simulink model "NLGC_4"  (R2017b)
settings: Solver=ode45  StartTime=0.0  StopTime=30  FixedStep=0.05  MaxStep=0.06  RelTol=1e-3  EnableMultiTasking=on
model workspace (MAT data in the model file):
  Sig = Simulink.Signal
  Sig.DataType = 'auto'
  Sig.Dimensions = -1
  Sig.DimensionsMode = 'auto'
  Sig.Complexity = 'auto'
  Sig.SampleTime = -1
  Sig.SamplingMode = 'auto'
undefined symbols (not defined in the file): IC, psi, quadModel, x, y, z
libraries: simulink x12, NLGCToolbox x11, sharedtransform x1
Description:
  | This is a configurable quadcopter simulation.
  | This Simulink model demonstates position control.
  | 
  | Additional quadcopter modeling and simulation materials available at:
  | github.com/dch33/Quad-Sim
  | 
  | Copyright (C) 2014 D. Hartman, K. Landis, S. Moreno, J. Kim, M. Mehrer
  | 
  | License:
  |     This program is free software: you can redistribute it and/or modify
  |     it under the terms of the GNU LESSER GENERAL PUBLIC LICENSE as published by
  |     the Free Software Foundation, either version 3 of the License, or
  |     (at your option) any later version.
  | 
  |     This program is distributed in the hope that it will be useful,
  |     but WITHOUT ANY WARRANTY; without even the implied warranty of
  |     MERCHANTABILITY or FITNESS FOR A PARTICULAR PURPOSE.  See the
  |     GNU General Public License for more details.
  | 
  |     You should have received a copy of the GNU LESSER GENERAL PUBLIC LICENSE
  |     along with this program.  If not, see <http://www.gnu.org/licenses/>.
settings Model: ModifiedComment=hoang -- Wed Apr 11 06:13:36 2018 -- Version 1.7  Creator=David Hartman  LastModifiedBy=hoang
settings Model: ModifiedHistory=|
  | hoang -- Wed Apr 11 06:13:36 2018 -- Version 1.7
  | 
  | hoang -- Wed Apr 11 04:36:33 2018 -- Version 1.6
  | 
  | davidhartman -- Fri Jun 06 22:59:54 2014 -- Version 1.5
settings DataIOCC: SaveFormat=Array  SignalLogging=off
settings OptimizationCC: DefaultParameterBehavior=Inlined  LifeSpan=inf
settings DebuggingCC: SolverPrmCheckMsg=warning  UniqueDataStoreMsg=warning  StateNameClashWarn=warning  StrictBusMsg=ErrorOnBusTreatedAsVector  SFUnexpectedBacktrackingDiag=warning  SFNoUnconditionalDefaultTransitionDiag=warning  SFExecutionAtInitializationDiag=none
settings HardwareCC: ProdBitPerPointer=32  ProdBitPerSizeT=32  ProdBitPerPtrDiffT=32  ProdLargestAtomicFloat=None  ProdIntDivRoundTo=Undefined  ProdEndianess=Unspecified  ProdWordSize=32  ProdHWDeviceType=32-bit Generic
settings ModelReferenceCC: PropagateSignalLabelsOutOfModel=off
settings CodeAppCC: StateflowObjectComments=on
settings GRTTargetCC: TargetLangStandard=C89/C90 (ANSI)  GeneratePreprocessorConditionals=Disable all
settings ConfigComp: CovMetricSettings=dw  CovHtmlReporting=on  CovSaveCumulativeToWorkspaceVar=on  CovSaveSingleToWorkspaceVar=on  CovExternalEMLEnable=off

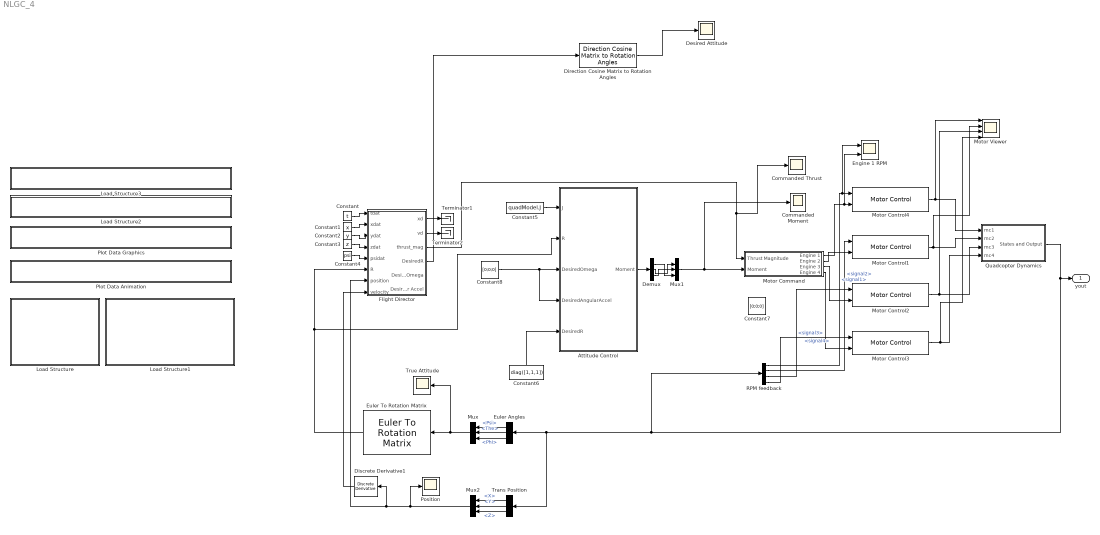
== system NLGC_4 ==
  Attitude Control : Subsystem  AncestorBlock=NLGCToolbox/Attitude Control  mask{kr=96, ko=1.25, Ts=1/60}
      mask prompts: kr "Attitude error gain (Kr)"; ko "Angular velocity error gain (Ko)"; Ts "Sampling Time (Ts)"
      mask init:
      | set_param(gcb, 'MaskSelfModifiable', 'on');
      settings: OpenFcn=set_param(gcbh,'LinkStatus','none');
  Commanded Thrust : Scope
  Commanded Moment : Scope
  Constant : Constant  Value=t
  Constant1 : Constant  Value=x
  Constant2 : Constant  Value=y
  Constant3 : Constant  Value=z
  Constant4 : Constant  Value=psi
  Constant5 : Constant  Value=quadModel.J
  Constant6 : Constant  Value=diag([1,1,1])
  Constant7 : Constant  Value=[0;0;0]
  Constant8 : Constant  Value=[0;0;0]
  Demux : Demux  Outputs=3
  Desired Attitude : Scope
  Direction Cosine Matrix to Rotation Angles : sharedtransform/Direction Cosine Matrix to Rotation Angles  rotationOrder=XYZ
      settings: SourceProductName=Aerospace Blockset  SourceProductBaseCode=AE
  Discrete Derivative1 : simulink/Discrete/Discrete Derivative  gainval=1.0  ICPrevScaledInput=[IC.X;IC.Y;IC.Z]*60  OutMin=[]  OutMax=[]  OutDataType=fixdt(1, 16)  OutScaling=2^-10  DoSatur=off
  Engine 1 RPM : Scope  NumInputPorts=2
  Euler Angles : BusSelector  OutputSignals=Psi,The,Phi
  Euler To Rotation Matrix : NLGCToolbox/Euler To Rotation Matrix
      settings: SourceProductName=Thinh - NLGC for Quadrotor
  Flight Director : Subsystem  AncestorBlock=NLGCToolbox/Flight Director  mask{Ts=1/60, kx=16, kv=5.6}
      mask prompts: Ts "Sampling Time (Ts)"; kx "Position Control Gain (kx)"; kv "Velocity Control Gain (kv)"
      settings: OpenFcn=set_param(gcbh,'LinkStatus','none');
  Load Structure : Subsystem
      settings: OpenFcn=|
      | uiopen('load')
      | if ((exist('IC')==1) && (exist('quadModel')==1) && (exist('path')==1))
      | set_param(bdroot, 'SimulationCommand', 'update')
      | end
      mask Display: fprintf('LOAD:\nTimeseries\nPath\nCommands,\nQuadcopter\nModel, Or\nInitial\nConditions');
  Load Structure1 : Subsystem
      settings: OpenFcn=|
      | if (exist('IC')==1 && exist('quadModel')==1 && exist('yout') && exist('tout'))
      | saveSimResults()
      | else
      | msgbox('No Data To Save!')
      | end
      mask Display: fprintf('SAVE:\nSimulation\nResults');
  Load Structure2 : Subsystem
      settings: OpenFcn=|
      | if exist('GUI_Modeling') == 2,
      | run('GUI_Modeling')
      | 
      | else
      | 
      | msgbox('The desired GUI must be first added to MATLABs path.')
      | 
      | end
      mask Display: fprintf('OPEN GUI: Build New \n Model');
  Load Structure3 : Subsystem
      settings: OpenFcn=|
      | if exist('GUI_IC') == 2,
      | run('GUI_IC')
      | 
      | else
      | 
      | msgbox('The desired GUI must be first added to MATLABs path.')
      | 
      | end
      mask Display: fprintf('OPEN GUI: Create Initial \n Conditions');
  Motor Command : Subsystem  AncestorBlock=NLGCToolbox/Motor Command  mask{Ct=quadModel.ct, dctcq=quadModel.dctcq}
      mask prompts: Ct "Force coefficient (Ct)"; dctcq "Moment coefficients matrix (dctcq)"
      settings: OpenFcn=set_param(gcbh,'LinkStatus','none');
  Motor Control{1..4} (4 alike) : NLGCToolbox/Motor Control  k=2.26  Km=quadModel.cr  Ts=1/60  T=quadModel.T  Rdt=100  Rdx=2  b=quadModel.b
      settings: SourceProductName=Thinh - NLGC for Quadrotor
  Motor Viewer : Scope  NumInputPorts=4
  Mux : Mux  Inputs=3
  Mux1 : Mux  Inputs=3
  Mux2 : Mux  Inputs=3
  Plot Data Animation : Subsystem
      settings: OpenFcn=|
      | if exist('QuadAnim4') == 2,
      |     if exist('yout')
      | 	run('QuadAnim4');
      |     else
      |     msgbox('Simulation must be run before data can be plotted.');
      |     end
      | else                                                                          msgbox('The desired GUI must be first added to MATLABs path.')
      | end
      mask Display: fprintf('OPEN GUI: Flight Animation')
  Plot Data Graphics : Subsystem
      settings: OpenFcn=|
      | if exist('yout')
      | yout = evalin('base', 'yout');
      | tout = evalin('base', 'tout');
      | quadPlots(yout, tout)
      | else
      | msgbox('Simulation must be run before data can be plotted.')
      | end
      mask Display: fprintf('OPEN PLOT: State Data')
  Position : Scope
  Quadcopter Dynamics : Subsystem
  RPM feedback : BusSelector  OutputSignals=mc and RPM.signal1,mc and RPM.signal2,mc and RPM.signal3,mc and RPM.signal4
  Terminator1 : Terminator
  Terminator2 : Terminator
  Trans Position : BusSelector  OutputSignals=X,Y,Z
  True Attitude : Scope
  yout : Outport
  wires:
  Quadcopter Dynamics/1(States and Output) -> RPM feedback/1, Trans Position/1, Euler Angles/1, yout/1
  Mux/1 -> Euler To Rotation Matrix/1, True Attitude/1
  Trans Position/3 -> Mux2/3  "<Z>"
  Mux2/1 -> Position/1, Flight Director/7(position), Discrete Derivative1/1
  Constant5/1 -> Attitude Control/1(J)
  Flight Director/3(thrust_mag) -> Motor Command/1(" Thrust Magnitude"), Commanded Thrust/1
  Motor Command/1(Engine 1) -> Motor Control4/2, Engine 1 RPM/2
  Motor Command/2(Engine 2) -> Motor Control1/2
  Motor Command/3(Engine 3) -> Motor Control2/2
  Motor Command/4(Engine 4) -> Motor Control3/2
  Motor Control4/1 -> Motor Viewer/1, Quadcopter Dynamics/1(mc1)
  Motor Control1/1 -> Motor Viewer/2, Quadcopter Dynamics/2(mc2)
  Motor Control3/1 -> Motor Viewer/4, Quadcopter Dynamics/4(mc4)
  RPM feedback/1 -> Motor Control4/1, Engine 1 RPM/1  "<signal1>"
  RPM feedback/2 -> Motor Control1/1  "<signal2>"
  RPM feedback/3 -> Motor Control2/1  "<signal3>"
  RPM feedback/4 -> Motor Control3/1  "<signal4>"
  Constant/1 -> Flight Director/1(tdat)
  Constant1/1 -> Flight Director/2(xdat)
  Discrete Derivative1/1 -> Flight Director/8(velocity)
  Direction Cosine Matrix to Rotation Angles/1 -> Desired Attitude/1
  Motor Control2/1 -> Motor Viewer/3, Quadcopter Dynamics/3(mc3)
  Trans Position/2 -> Mux2/2  "<Y>"
  Trans Position/1 -> Mux2/1  "<X>"
  Euler Angles/1 -> Mux/1  "<Psi>"
  Euler Angles/2 -> Mux/2  "<The>"
  Euler Angles/3 -> Mux/3  "<Phi>"
  Flight Director/4(DesiredR) -> Direction Cosine Matrix to Rotation Angles/1
  Constant2/1 -> Flight Director/3(ydat)
  Constant3/1 -> Flight Director/4(zdat)
  Constant4/1 -> Flight Director/5(psidat)
  Flight Director/1(xd) -> Terminator1/1
  Flight Director/2(vd) -> Terminator2/1
  Attitude Control/1(Moment) -> Demux/1
  Mux1/1 -> Commanded Moment/1, Motor Command/2(Moment)
  Constant8/1 -> Attitude Control/4(DesiredAngularAccel), Attitude Control/3(DesiredOmega)
  ? -> ?
  Euler To Rotation Matrix/1 -> Attitude Control/2(R), Flight Director/6(R)
  Constant6/1 -> Attitude Control/5(DesiredR)
  Demux/1 -> Mux1/3
  Demux/3 -> Mux1/1
  Demux/2 -> Mux1/2

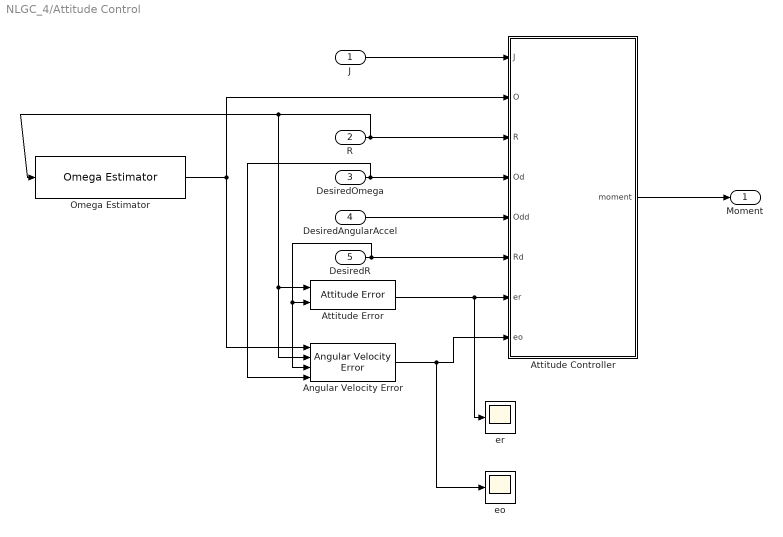
== system NLGC_4/Attitude Control ==
  J : Inport
  R : Inport  Port=2
  DesiredOmega : Inport  Port=3
  DesiredAngularAccel : Inport  Port=4
  DesiredR : Inport  Port=5
  Angular Velocity Error : NLGCToolbox/Angular Velocity Error
      settings: SourceProductName=Thinh - NLGC for Quadrotor
  Attitude Controller : MATLAB Function  TreatAsAtomicUnit=on
  Attitude Error : NLGCToolbox/Attitude Error
      settings: SourceProductName=Thinh - NLGC for Quadrotor
  Omega Estimator : NLGCToolbox/Omega Estimator  Ts=Ts
      settings: SourceProductName=Thinh - NLGC for Quadrotor
  eo : Scope
  er : Scope
  Moment : Outport
  wires:
  Angular Velocity Error/1 -> eo/1, Attitude Controller/8(eo)
  Attitude Error/1 -> er/1, Attitude Controller/7(er)
  J/1 -> Attitude Controller/1(J)
  Omega Estimator/1 -> Angular Velocity Error/1, Attitude Controller/2(O)
  R/1 -> Attitude Controller/3(R), Omega Estimator/1, Attitude Error/1, Angular Velocity Error/2
  DesiredOmega/1 -> Attitude Controller/4(Od), Angular Velocity Error/4
  DesiredAngularAccel/1 -> Attitude Controller/5(Odd)
  DesiredR/1 -> Attitude Controller/6(Rd), Attitude Error/2, Angular Velocity Error/3
  Attitude Controller/1(moment) -> Moment/1

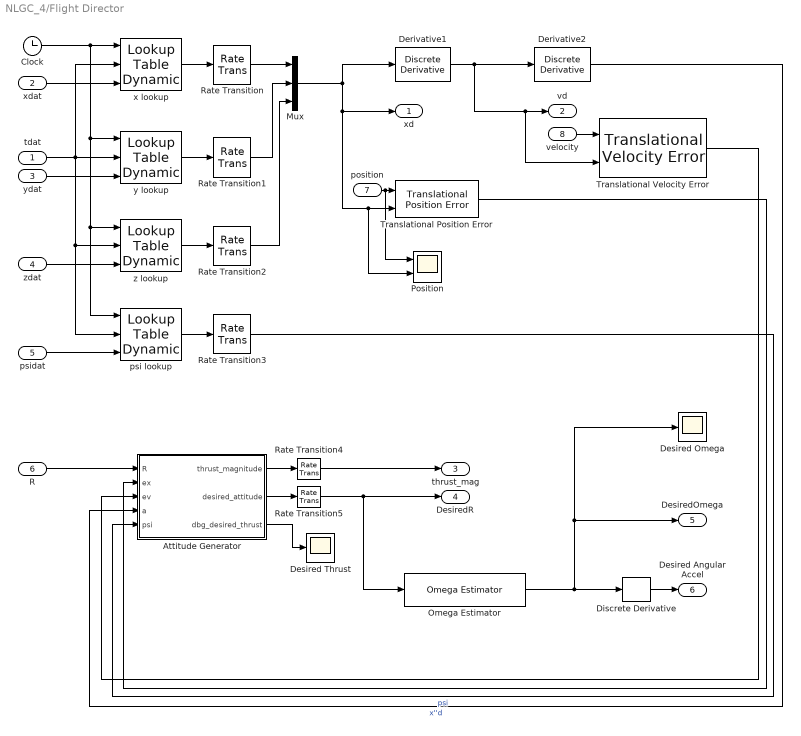
== system NLGC_4/Flight Director ==
  tdat : Inport
  xdat : Inport  Port=2
  ydat : Inport  Port=3
  zdat : Inport  Port=4
  psidat : Inport  Port=5
  R : Inport  Port=6
  position : Inport  Port=7
  velocity : Inport  Port=8
  Attitude Generator : MATLAB Function  TreatAsAtomicUnit=on
  Clock : Clock
  Derivative1 : simulink/Discrete/Discrete Derivative  gainval=1.0  ICPrevScaledInput=[0;0;3]*60  OutMin=[]  OutMax=[]  OutDataType=fixdt(1, 16)  OutScaling=2^-10  DoSatur=off
  Derivative2 : simulink/Discrete/Discrete Derivative  gainval=1.0  ICPrevScaledInput=0.0  OutMin=[]  OutMax=[]  OutDataType=fixdt(1, 16)  OutScaling=2^-10  DoSatur=off
  Desired Omega : Scope
  Desired Thrust : Scope
  Discrete Derivative : simulink/Discrete/Discrete Derivative  gainval=1.0  ICPrevScaledInput=0.0  OutMin=[]  OutMax=[]  OutDataType=fixdt(1, 16)  OutScaling=2^-10  DoSatur=off
  Mux : Mux  Inputs=3
  Omega Estimator : NLGCToolbox/Omega Estimator  Ts=Ts
      settings: SourceProductName=Thinh - NLGC for Quadrotor
  Position : Scope  NumInputPorts=2
  Rate Transition{,1..5} (6 alike) : RateTransition  OutPortSampleTime=Ts
  Translational Position Error : NLGCToolbox/Translational Position Error
      settings: SourceProductName=Thinh - NLGC for Quadrotor
  Translational Velocity Error : NLGCToolbox/Translational Velocity Error
      settings: SourceProductName=Thinh - NLGC for Quadrotor
  psi lookup : simulink/Lookup Tables/Lookup Table Dynamic  LookUpMeth=Interpolation-Use End Values  OutDataType=fixdt('double')  OutScaling=[]  OutputDataTypeScalingMode=Specify via dialog  OutDataTypeStr=double  DoSatur=off
      settings: SourceProductName=Simulink
  x lookup : simulink/Lookup Tables/Lookup Table Dynamic  LookUpMeth=Interpolation-Use End Values  OutDataType=fixdt('double')  OutScaling=[]  OutputDataTypeScalingMode=Specify via dialog  OutDataTypeStr=double  DoSatur=off
      settings: SourceProductName=Simulink
  y lookup : simulink/Lookup Tables/Lookup Table Dynamic  LookUpMeth=Interpolation-Use End Values  OutDataType=fixdt('double')  OutScaling=[]  OutputDataTypeScalingMode=Specify via dialog  OutDataTypeStr=double  DoSatur=off
      settings: SourceProductName=Simulink
  z lookup : simulink/Lookup Tables/Lookup Table Dynamic  LookUpMeth=Interpolation-Use End Values  OutDataType=fixdt('double')  OutScaling=[]  OutputDataTypeScalingMode=Specify via dialog  OutDataTypeStr=double  DoSatur=off
      settings: SourceProductName=Simulink
  xd : Outport
  vd : Outport  Port=2
  thrust_mag : Outport  Port=3
  DesiredR : Outport  Port=4
  DesiredOmega : Outport  Port=5
  Desired Angular Accel : Outport  Port=6
  wires:
  Omega Estimator/1 -> Discrete Derivative/1, DesiredOmega/1, Desired Omega/1
  velocity/1 -> Translational Velocity Error/1
  psidat/1 -> psi lookup/3
  Translational Velocity Error/1 -> Attitude Generator/3(ev)
  Translational Position Error/1 -> Attitude Generator/2(ex)
  Mux/1 -> Derivative1/1, Position/2, Translational Position Error/2, xd/1
  Rate Transition4/1 -> thrust_mag/1
  Rate Transition5/1 -> DesiredR/1, Omega Estimator/1
  Discrete Derivative/1 -> Desired Angular Accel/1
  R/1 -> Attitude Generator/1(R)
  Attitude Generator/2(desired_attitude) -> Rate Transition5/1
  Attitude Generator/1(thrust_magnitude) -> Rate Transition4/1
  Rate Transition3/1 -> Attitude Generator/5(psi)  "psi"
  Derivative2/1 -> Attitude Generator/4(a)  "x''d"
  psi lookup/1 -> Rate Transition3/1
  Derivative1/1 -> Derivative2/1, vd/1, Translational Velocity Error/2
  Rate Transition2/1 -> Mux/3
  Rate Transition1/1 -> Mux/2
  Rate Transition/1 -> Mux/1
  z lookup/1 -> Rate Transition2/1
  y lookup/1 -> Rate Transition1/1
  x lookup/1 -> Rate Transition/1
  zdat/1 -> z lookup/3
  ydat/1 -> y lookup/3
  xdat/1 -> x lookup/3
  Clock/1 -> x lookup/1, y lookup/1, z lookup/1, psi lookup/1
  tdat/1 -> y lookup/2, x lookup/2, z lookup/2, psi lookup/2
  Attitude Generator/3(dbg_desired_thrust) -> Desired Thrust/1
  position/1 -> Position/1, Translational Position Error/1

== system NLGC_4/Load Structure ==

== system NLGC_4/Load Structure1 ==

== system NLGC_4/Load Structure2 ==

== system NLGC_4/Load Structure3 ==

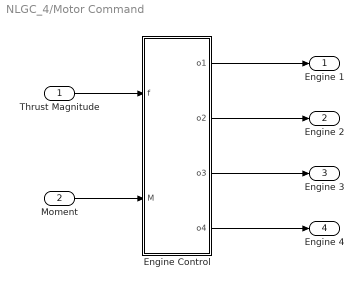
== system NLGC_4/Motor Command ==
  " Thrust Magnitude" : Inport
  Moment : Inport  Port=2
  Engine Control : MATLAB Function  TreatAsAtomicUnit=on
  Engine 1 : Outport
  Engine 2 : Outport  Port=2
  Engine 3 : Outport  Port=3
  Engine 4 : Outport  Port=4
  wires:
  Engine Control/4(o4) -> Engine 4/1
  Engine Control/3(o3) -> Engine 3/1
  Engine Control/2(o2) -> Engine 2/1
  Engine Control/1(o1) -> Engine 1/1
  Moment/1 -> Engine Control/2(M)
  " Thrust Magnitude"/1 -> Engine Control/1(f)

== system NLGC_4/Plot Data Animation ==

== system NLGC_4/Plot Data Graphics ==

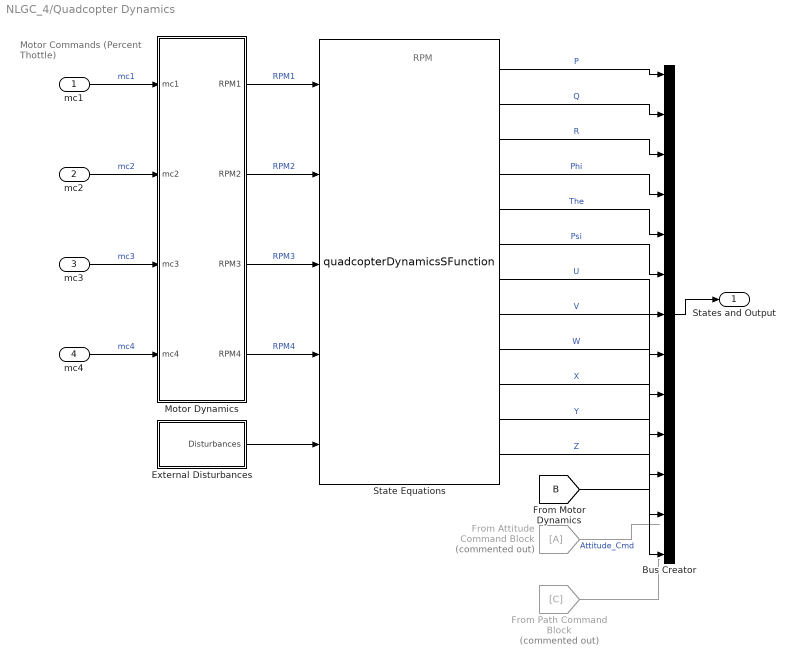
== system NLGC_4/Quadcopter Dynamics ==
  note: RPM
  note: Motor Commands
      | (Percent Thottle)
  mc1 : Inport
  mc2 : Inport  Port=2
  mc3 : Inport  Port=3
  mc4 : Inport  Port=4
  Bus Creator : BusCreator  Inputs=P,Q,R,Phi,The,Psi,U,V,W,X,Y,Z,mc and RPM
  External Disturbances : Subsystem
  From Attitude Command Block : From  Commented=on  TagVisibility=global
  From Path Command Block : From  Commented=on  GotoTag=C  TagVisibility=global
  Motor Dynamics : Subsystem
  State Equations : M-S-Function  FunctionName=quadcopterDynamicsSFunction  Parameters=quadModel, IC
      mask Display:
      | port_label('input', 1, 'RPM1')
      | port_label('input', 2, 'RPM2')
      | port_label('input', 3, 'RPM3')
      | port_label('input', 4, 'RPM4')
      | port_label('input', 5, 'Disturbances')
      | port_label('output', 1, 'P')
      | port_label('output', 2, 'Q')
      | port_label('output', 3, 'R')
      | port_label('output', 4, 'Phi')
      | port_label('output', 5, 'The')
      | port_label('output', 6, 'Psi')
      | port_label('output', 7, 'U')
      | port_label('output', 8, 'V')
      | port_label('output', 9, 'W')
      | port_label('output', 10, 'X')
      | port_label('output', 11, 'Y')
      | port_label('output', 12, 'Z')
  States and Output : Outport
  wires:
  State Equations/1 -> Bus Creator/1  "P"
  State Equations/2 -> Bus Creator/2  "Q"
  State Equations/3 -> Bus Creator/3  "R"
  State Equations/4 -> Bus Creator/4  "Phi"
  State Equations/5 -> Bus Creator/5  "The"
  State Equations/6 -> Bus Creator/6  "Psi"
  State Equations/7 -> Bus Creator/7  "U"
  State Equations/8 -> Bus Creator/8  "V"
  State Equations/9 -> Bus Creator/9  "W"
  State Equations/10 -> Bus Creator/10  "X"
  State Equations/11 -> Bus Creator/11  "Y"
  State Equations/12 -> Bus Creator/12  "Z"
  Bus Creator/1 -> States and Output/1
  Motor Dynamics/1(RPM1) -> State Equations/1  "RPM1"
  Motor Dynamics/2(RPM2) -> State Equations/2  "RPM2"
  Motor Dynamics/3(RPM3) -> State Equations/3  "RPM3"
  Motor Dynamics/4(RPM4) -> State Equations/4  "RPM4"
  mc1/1 -> Motor Dynamics/1(mc1)  "mc1"
  mc4/1 -> Motor Dynamics/4(mc4)  "mc4"
  mc3/1 -> Motor Dynamics/3(mc3)  "mc3"
  mc2/1 -> Motor Dynamics/2(mc2)  "mc2"
  External Disturbances/1("Disturbances ") -> State Equations/5
  From Attitude Command Block/1 -> ?  "Attitude_Cmd"
  [B] -> Bus Creator/13
  From Path Command Block/1 -> ?

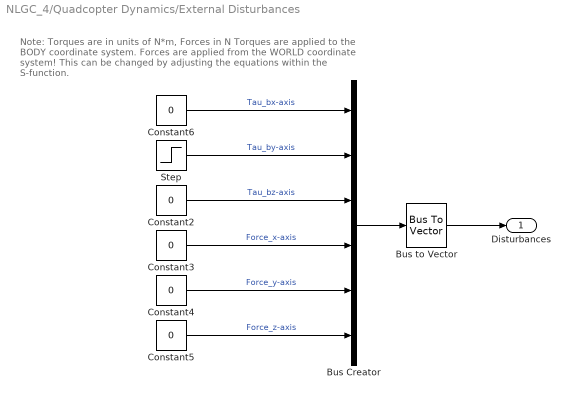
== system NLGC_4/Quadcopter Dynamics/External Disturbances ==
  note: Note: Torques are in units of N*m, Forces in N
      | Torques are applied to the BODY coordinate system.
      | Forces are applied from the WORLD coordinate system!
      | This can be changed by adjusting the equations within the S-function.
  Bus Creator : BusCreator  Inputs=6
  Bus to Vector : BusToVector
  Constant{2..6} (5 alike) : Constant  Value=0
  Step : Step  After=0  SampleTime=0
  "Disturbances " : Outport
  wires:
  Bus to Vector/1 -> "Disturbances "/1
  Bus Creator/1 -> Bus to Vector/1
  Constant6/1 -> Bus Creator/1  "Tau_bx-axis"
  Step/1 -> Bus Creator/2  "Tau_by-axis"
  Constant2/1 -> Bus Creator/3  "Tau_bz-axis"
  Constant3/1 -> Bus Creator/4  "Force_x-axis"
  Constant4/1 -> Bus Creator/5  "Force_y-axis"
  Constant5/1 -> Bus Creator/6  "Force_z-axis"

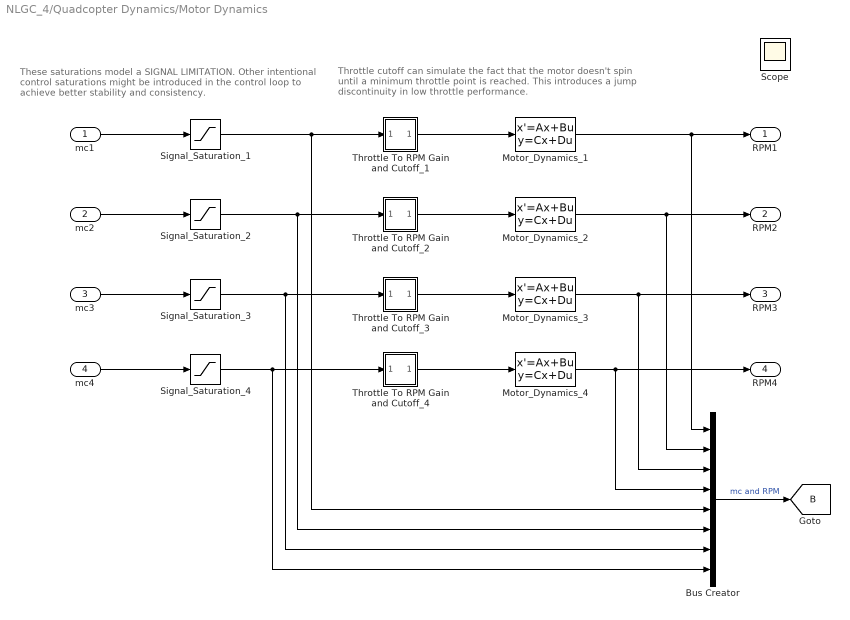
== system NLGC_4/Quadcopter Dynamics/Motor Dynamics ==
  note: Throttle cutoff can simulate the fact that the motor doesn't
      | spin until a minimum throttle point is reached. This introduces
      | a jump discontinuity in low throttle performance.
  note: These saturations model a SIGNAL LIMITATION.
      | Other intentional control saturations might be introduced in the
      | control loop to achieve better stability and consistency.
  mc1 : Inport
  mc2 : Inport  Port=2
  mc3 : Inport  Port=3
  mc4 : Inport  Port=4
  Bus Creator : BusCreator  Inputs=8
  Motor_Dynamics_1 : StateSpace  A=-1/quadModel.T  C=1/quadModel.T  D=0  InitialCondition=IC.w1*quadModel.T
  Motor_Dynamics_2 : StateSpace  A=-1/quadModel.T  C=1/quadModel.T  D=0  InitialCondition=IC.w2*quadModel.T
  Motor_Dynamics_3 : StateSpace  A=-1/quadModel.T  C=1/quadModel.T  D=0  InitialCondition=IC.w3*quadModel.T
  Motor_Dynamics_4 : StateSpace  A=-1/quadModel.T  C=1/quadModel.T  D=0  InitialCondition=IC.w4*quadModel.T
  Scope : Scope
  Signal_Saturation_{1..4} (4 alike) : Saturate  UpperLimit=100  LowerLimit=0
  Throttle To RPM Gain and Cutoff_1 : Subsystem
  Throttle To RPM Gain and Cutoff_2 : Subsystem
  Throttle To RPM Gain and Cutoff_3 : Subsystem
  Throttle To RPM Gain and Cutoff_4 : Subsystem
  RPM1 : Outport
  RPM2 : Outport  Port=2
  RPM3 : Outport  Port=3
  RPM4 : Outport  Port=4
  tag scope: B=global
  wires:
  mc1/1 -> Signal_Saturation_1/1
  mc4/1 -> Signal_Saturation_4/1
  mc2/1 -> Signal_Saturation_2/1
  mc3/1 -> Signal_Saturation_3/1
  Signal_Saturation_1/1 -> Bus Creator/5, Throttle To RPM Gain and Cutoff_1/1(In5)
  Signal_Saturation_2/1 -> Bus Creator/6, Throttle To RPM Gain and Cutoff_2/1(In5)
  Signal_Saturation_3/1 -> Bus Creator/7, Throttle To RPM Gain and Cutoff_3/1(In5)
  Signal_Saturation_4/1 -> Bus Creator/8, Throttle To RPM Gain and Cutoff_4/1(In5)
  Throttle To RPM Gain and Cutoff_1/1(Out5) -> Motor_Dynamics_1/1
  Throttle To RPM Gain and Cutoff_2/1(Out5) -> Motor_Dynamics_2/1
  Throttle To RPM Gain and Cutoff_3/1(Out5) -> Motor_Dynamics_3/1
  Throttle To RPM Gain and Cutoff_4/1(Out5) -> Motor_Dynamics_4/1
  Motor_Dynamics_1/1 -> Bus Creator/1, RPM1/1
  Motor_Dynamics_2/1 -> Bus Creator/2, RPM2/1
  Motor_Dynamics_3/1 -> Bus Creator/3, RPM3/1
  Motor_Dynamics_4/1 -> Bus Creator/4, RPM4/1
  Bus Creator/1 -> [B]  "mc and RPM"

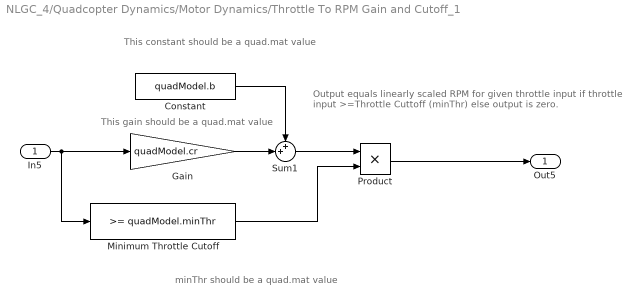
== system NLGC_4/Quadcopter Dynamics/Motor Dynamics/Throttle To RPM Gain and Cutoff_1 ==
  note: minThr should be a quad.mat value
  note: This gain should be a quad.mat value
  note: This constant should be a quad.mat value
  note: Output equals linearly scaled RPM
      | for given throttle input if throttle input >=Throttle Cuttoff (minThr)
      | else output is zero.
  In5 : Inport
  Constant : Constant  Value=quadModel.b
  Gain : Gain  Gain=quadModel.cr
  Minimum Throttle Cutoff : simulink/Logic and Bit Operations/Compare To Constant  relop=>=  const=quadModel.minThr  OutDataTypeStr=uint8
  Product : Product
  Sum1 : Sum  Inputs=++|
  Out5 : Outport
  wires:
  Minimum Throttle Cutoff/1 -> Product/2
  Product/1 -> Out5/1
  In5/1 -> Gain/1, Minimum Throttle Cutoff/1
  Gain/1 -> Sum1/2
  Sum1/1 -> Product/1
  Constant/1 -> Sum1/1

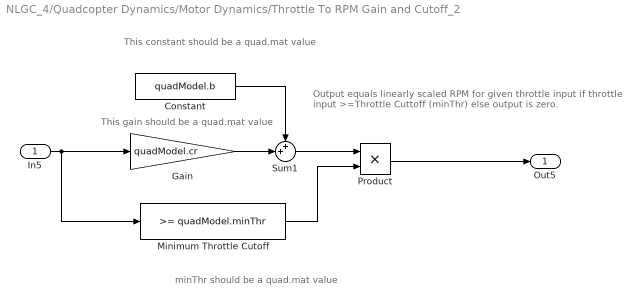
== system NLGC_4/Quadcopter Dynamics/Motor Dynamics/Throttle To RPM Gain and Cutoff_2 ==
  note: minThr should be a quad.mat value
  note: This gain should be a quad.mat value
  note: This constant should be a quad.mat value
  note: Output equals linearly scaled RPM
      | for given throttle input if throttle input >=Throttle Cuttoff (minThr)
      | else output is zero.
  In5 : Inport
  Constant : Constant  Value=quadModel.b
  Gain : Gain  Gain=quadModel.cr
  Minimum Throttle Cutoff : simulink/Logic and Bit Operations/Compare To Constant  relop=>=  const=quadModel.minThr  OutDataTypeStr=uint8
  Product : Product
  Sum1 : Sum  Inputs=++|
  Out5 : Outport
  wires:
  Minimum Throttle Cutoff/1 -> Product/2
  Product/1 -> Out5/1
  In5/1 -> Gain/1, Minimum Throttle Cutoff/1
  Gain/1 -> Sum1/2
  Sum1/1 -> Product/1
  Constant/1 -> Sum1/1

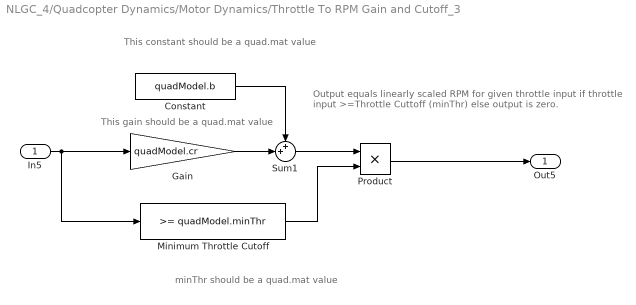
== system NLGC_4/Quadcopter Dynamics/Motor Dynamics/Throttle To RPM Gain and Cutoff_3 ==
  note: minThr should be a quad.mat value
  note: This gain should be a quad.mat value
  note: This constant should be a quad.mat value
  note: Output equals linearly scaled RPM
      | for given throttle input if throttle input >=Throttle Cuttoff (minThr)
      | else output is zero.
  In5 : Inport
  Constant : Constant  Value=quadModel.b
  Gain : Gain  Gain=quadModel.cr
  Minimum Throttle Cutoff : simulink/Logic and Bit Operations/Compare To Constant  relop=>=  const=quadModel.minThr  OutDataTypeStr=uint8
  Product : Product
  Sum1 : Sum  Inputs=++|
  Out5 : Outport
  wires:
  Minimum Throttle Cutoff/1 -> Product/2
  Product/1 -> Out5/1
  In5/1 -> Gain/1, Minimum Throttle Cutoff/1
  Gain/1 -> Sum1/2
  Sum1/1 -> Product/1
  Constant/1 -> Sum1/1

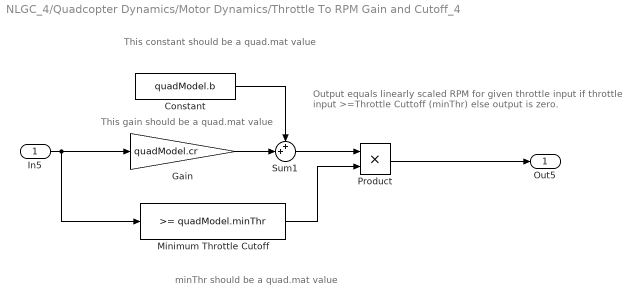
== system NLGC_4/Quadcopter Dynamics/Motor Dynamics/Throttle To RPM Gain and Cutoff_4 ==
  note: minThr should be a quad.mat value
  note: This gain should be a quad.mat value
  note: This constant should be a quad.mat value
  note: Output equals linearly scaled RPM
      | for given throttle input if throttle input >=Throttle Cuttoff (minThr)
      | else output is zero.
  In5 : Inport
  Constant : Constant  Value=quadModel.b
  Gain : Gain  Gain=quadModel.cr
  Minimum Throttle Cutoff : simulink/Logic and Bit Operations/Compare To Constant  relop=>=  const=quadModel.minThr  OutDataTypeStr=uint8
  Product : Product
  Sum1 : Sum  Inputs=++|
  Out5 : Outport
  wires:
  Minimum Throttle Cutoff/1 -> Product/2
  Product/1 -> Out5/1
  In5/1 -> Gain/1, Minimum Throttle Cutoff/1
  Gain/1 -> Sum1/2
  Sum1/1 -> Product/1
  Constant/1 -> Sum1/1

== matlab function NLGC_4/Flight Director/Attitude Generator ==
  data: R input size=[3 3]; thrust_magnitude output size=1; ex input size=[3 1]; ev input size=[3 1]; a input size=[3 1]; psi input size=1; desired_attitude output size=[3 3]; kx parameter; kv parameter; quadModel parameter; dbg_desired_thrust output
function [thrust_magnitude,desired_attitude,dbg_desired_thrust] = fcn(R,ex,ev,a,psi,kx,kv,quadModel) % R: b->i

e3 = [0 0 1]';

if (norm(a)>100) % Fuse for large intial derivatives
    a = [0;0;0];
end 

desired_thrust = - kx*ex - kv*ev + quadModel.mass*quadModel.g*e3 + quadModel.mass*a;
dbg_desired_thrust = desired_thrust;

% Desired Attitude Calculation
z_direction = desired_thrust/norm(desired_thrust); % b3, from [0 0 1]'
x_direction = findDirection(psi, z_direction, 0); % b1, from [1 0 0]'
y_direction = hat(z_direction)*x_direction; % b2, from [0 1 0]'
desired_attitude = [x_direction y_direction z_direction]; % b->i, since R[1 0 0]' = x_direction => RI = R, thus it eats a body vector and returns an inertial vector
thrust_magnitude = norm(desired_thrust) * (e3'*R'*desired_attitude*e3);

end

% Function to find Promoted Direction Vector
function y = findDirection(psi,thrust_direction,initial_pitch)
Rpsi = tangle2dcm(psi,initial_pitch,0); % i->b
ddv = Rpsi'*[1 0 0]'; % Provisional Desired Direction Vector (DDV)
pdv = - (hat(thrust_direction) * (hat(thrust_direction) * ddv)); % Promoted Direction Vector (PDV)
y = pdv/norm(pdv);
end

== matlab function NLGC_4/Attitude Control/Attitude Controller ==
  data: J input size=[3 3]; moment output size=[3 1]; O input size=[3 1]; R input size=[3 3]; Od input size=[3 1]; Odd input size=[3 1]; Rd input size=[3 3]; er input size=[3 1]; eo input size=[3 1]; kr parameter; ko parameter
function moment = fcn(J,O,R,Od,Odd,Rd,er,eo,kr, ko)
moment = hat(O)*(J*O) - J*(hat(O)*R'*Rd*Od - R'*Rd*Odd + kr * er + ko * eo);

== matlab function NLGC_4/Motor Command/Engine Control ==
  data: f input size=1; o1 output size=1; M input size=[3 1]; o2 output size=1; o3 output size=1; o4 output size=1; Ct parameter; dctcq parameter size=[3 4]
function [o1,o2,o3,o4] = fcn(f,M,Ct,dctcq)
force = [f; M];
gamma = [Ct Ct Ct Ct;
    dctcq];
omega_sq = gamma\force;
omega=zeros(4,1);
for i=1:4
    if omega_sq(i)>0
        omega(i)=sqrt(omega_sq(i));
    else
        omega(i)=0;
    end
end
o1=omega(1);
o2=omega(2);
o3=omega(3);
o4=omega(4);
